simulink library "tpl"  (Simulink 8.1)
settings: Solver=ode1  StartTime=0.0  StopTime=Inf  FixedStep=0.001  RelTol=1e-3
PostLoadFcn:
  | , if any(exist('dsrtsu_mdlpostloadfcn', 'file') == [2, 3, 6]), try dsrtsu_mdlpostloadfcn('Execute', bdroot); catch fprintf('Error in PostLoadFcn (dsrtsu_mdlpostloadfcn) for model "%s":\n %s\n', bdroot, lasterr); end, end,
undefined symbols (not defined in the file or in its folder): KACC_EngTqMaxMargin_Nm, KACC_EngTqMinMargin_Nm
libraries: hcu_lib x1
settings Model: DSRTSU_INTERNAL_RTI_VER=450  DSRTSU_INTERNAL_RTI_TYPE=rti1401  RTICANMMDATA=struct('GeneralSetupData',struct('modelroot','D:\Projects\ELN150201\Repositories\Taiwan\trunk\AdasDragon\software\sw_development\arch\app\acc','generalsettings',struct('filesettings',struct('destfolder',struct('Name','RTICANMM_FILES','Check',1),'buildfolder',struct('Name','.','Check',1),'AbsDestfolder',struct('Name','D:\Projects\ELN150201\Repositories\Taiwan\trunk\AdasDragon\software\sw_development\arch\app\acc\RTICANMM_FILES'),'AbsBuildfolder',struct('Name','D:\Projects\ELN150201\Repositories\Taiwan\trunk\AdasDragon\software\sw_development\arch\app\acc'))),'options',struct('addpaths',1,'rmpaths',1,'addtrcexclusion',logical(1),'cannavigator',struct('checkmonitoring',0),'show_usrtrc',0,'use_usrtrc',0),'advanced',struct('options',[1 1 1 1 1 1 1 1 1 1 1 1 1 1 1 1 1 1 1 1 1 1 1 1 1 1 1 1 1 1 1 1 1 1 1 1 1 1 1 1 1 1 1 1 1 1 1 1 1 1 1 1 1 1 1 1 1 1 1 1 1 1 1 1 1 1 1 1 1 1 1 1 1 1 1 1 1 1 1 1 1 1 1 1 1 1 1 1 1 1 1 1 1 1 1 1 1 1 1 1]),'MPSetup',{{}},'modelname','Copy_of_scc','block','Copy_of_scc'))  DSRTSU_INTERNAL_RTIFPGA=40  Creator=AT015411  LastModifiedBy=AT015086

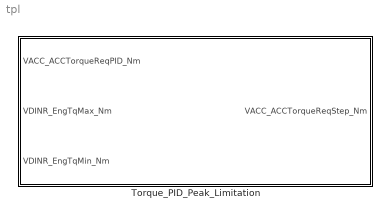
== system tpl ==
  Torque_PID_Peak_Limitation : Subsystem

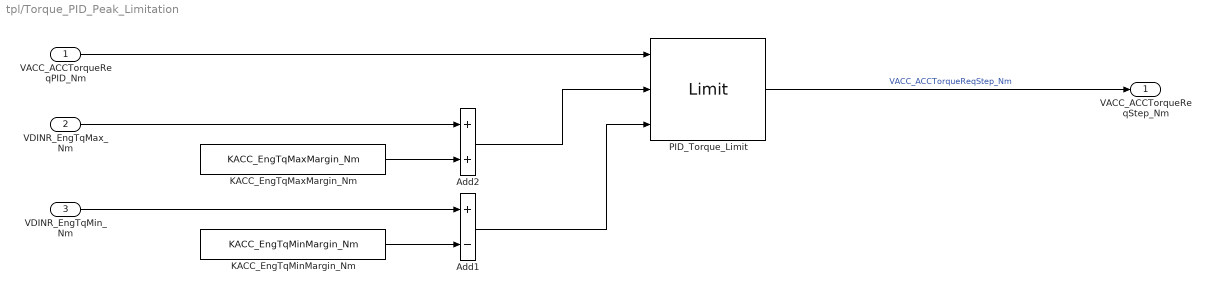
== system tpl/Torque_PID_Peak_Limitation ==
  VACC_ACCTorqueReqPID_Nm : Inport
  VDINR_EngTqMax_Nm : Inport  Port=2
  VDINR_EngTqMin_Nm : Inport  Port=3
  Add1 : Sum  Inputs=+-
  Add2 : Sum
  KACC_EngTqMaxMargin_Nm : Constant  Value=KACC_EngTqMaxMargin_Nm
  KACC_EngTqMinMargin_Nm : Constant  Value=KACC_EngTqMinMargin_Nm
  PID_Torque_Limit : hcu_lib/Limit  SystemSampleTime=-1
  VACC_ACCTorqueReqStep_Nm : Outport
  wires:
  Add2/1 -> PID_Torque_Limit/2
  VACC_ACCTorqueReqPID_Nm/1 -> PID_Torque_Limit/1
  Add1/1 -> PID_Torque_Limit/3
  VDINR_EngTqMin_Nm/1 -> Add1/1
  VDINR_EngTqMax_Nm/1 -> Add2/1
  KACC_EngTqMinMargin_Nm/1 -> Add1/2
  KACC_EngTqMaxMargin_Nm/1 -> Add2/2
  PID_Torque_Limit/1 -> VACC_ACCTorqueReqStep_Nm/1  "VACC_ACCTorqueReqStep_Nm"
